simulink model "DYNctl_ver4_etud_obfusc"  (R2021b)
settings: Solver=ode45  StartTime=0.0  StopTime=tfin  FixedStep=0.001  RelTol=1e-09  EnableMultiTasking=on
values from neighbouring files (symbols this model uses):
  A_lineaire = [ ... (first row only)    [equation_lineaire.m]
  Ax_e = 0    [Valeur_Equilibre.m]
  Ay_e = 0    [Valeur_Equilibre.m]
  B_lineaire = [ ... (first row only)    [equation_lineaire.m]
  C_lineaire = [ ... (first row only)    [equation_lineaire.m]
  C_variable_etat = eye(13,13)    [equation_lineaire.m]
  D_lineaire = zeros(7,3)    [equation_lineaire.m]
  D_variable_etat = zeros(13,3)    [equation_lineaire.m]
  Ia_e = i_A    [Valeur_Equilibre.m]
  Ib_e = i_B    [Valeur_Equilibre.m]
  Ic_e = i_C    [Valeur_Equilibre.m]
  Px_e = Px_sphere    [Valeur_Equilibre.m]
  Py_e = Py_sphere    [Valeur_Equilibre.m]
  Pz_e = Pz_plaque    [Valeur_Equilibre.m]
  Va_e = RR*Ia_e    [Valeur_Equilibre.m]
  Vb_e = RR*Ib_e    [Valeur_Equilibre.m]
  Vc_e = RR*Ic_e    [Valeur_Equilibre.m]
  Vx_e = 0    [Valeur_Equilibre.m]
  Vy_e = 0    [Valeur_Equilibre.m]
  Vz_e = 0    [Valeur_Equilibre.m]
  Wx_e = 0    [Valeur_Equilibre.m]
  Wy_e = 0    [Valeur_Equilibre.m]
  zD_e = Pz_plaque - XD*Ay_eq + YD*Ax_eq    [Valeur_Equilibre.m]
  zE_e = Pz_plaque - XE*Ay_eq + YE*Ax_eq    [Valeur_Equilibre.m]
  zF_e = Pz_plaque - XF*Ay_eq + YF*Ax_eq    [Valeur_Equilibre.m]
settings Model: Creator=delafontaine  LastModifiedBy=alexi
settings SolverCC: AlgebraicLoopSolver=LineSearch
settings DataIOCC: LimitDataPoints=on  SaveFormat=Array  SignalLoggingSaveFormat=ModelDataLogs  ReturnWorkspaceOutputs=off
settings OptimizationCC: LifeSpan=inf
settings DebuggingCC: UnderspecifiedInitializationDetection=Classic  MergeDetectMultiDrivingBlocksExec=none  MultiTaskDSMMsg=warning  MultiTaskCondExecSysMsg=none  SFUnexpectedBacktrackingDiag=warning  SFNoUnconditionalDefaultTransitionDiag=warning  SFExecutionAtInitializationDiag=none  SFMachineParentedDataDiag=warning  ArithmeticOperatorsInVariantConditions=warning
settings HardwareCC: ProdBitPerPointer=32  ProdBitPerSizeT=32  ProdBitPerPtrDiffT=32  ProdLargestAtomicFloat=None  ProdIntDivRoundTo=Undefined  ProdEndianess=Unspecified  ProdWordSize=32  ProdHWDeviceType=32-bit Generic
settings ModelReferenceCC: PropagateSignalLabelsOutOfModel=off
settings SFSimCC: SimUseLocalCustomCode=off  CustomCodeUndefinedFunction=UseInterfaceOnly
settings RTWCC: RTWUseLocalCustomCode=off
settings CodeAppCC: StateflowObjectComments=on
settings GRTTargetCC: TargetLangStandard=C89/C90 (ANSI)
settings ConfigComp: CovMetricSettings=dw  CovSaveCumulativeToWorkspaceVar=on  CovSaveSingleToWorkspaceVar=on  CovExternalEMLEnable=off  CovSFcnEnable=off

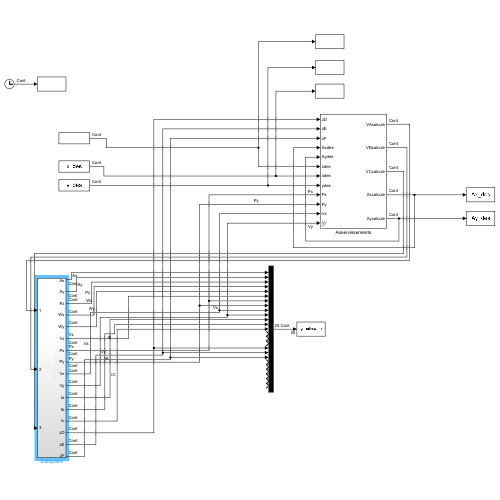
[thumbnail: Simulink's stored preview of the top-level diagram]
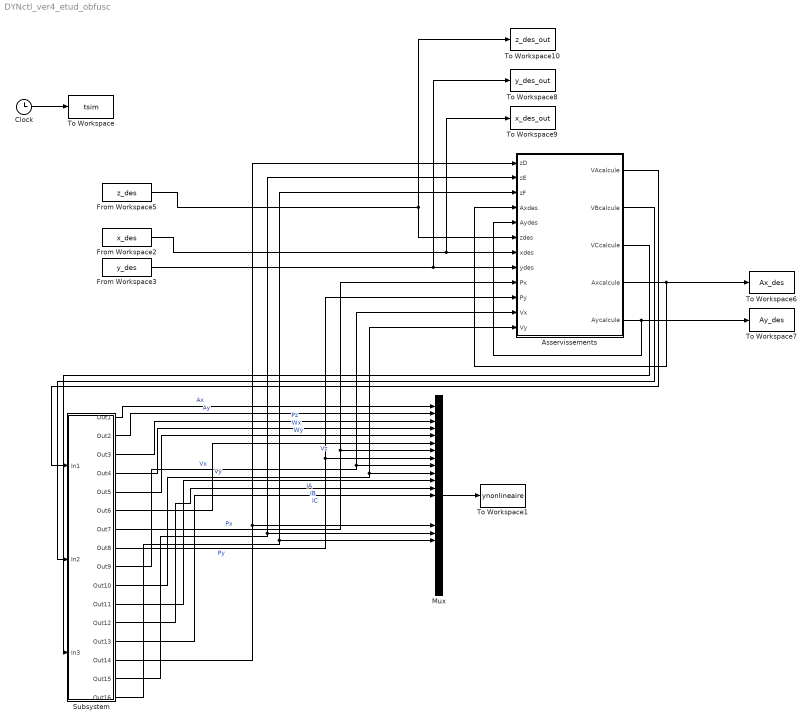
== system DYNctl_ver4_etud_obfusc ==
  Asservissements : Subsystem
      mask help: Simulink:masks:GenSFuncDesc_MD
      mask Help: eval('feval(''rtwprivate'',''rtwhelpview'',''rtw_sfcn_block'')');
  Clock : Clock
  From Workspace2 : FromWorkspace  VariableName=x_des  Interpolate=off  OutputAfterFinalValue=Holding final value
  From Workspace3 : FromWorkspace  VariableName=y_des  Interpolate=off  OutputAfterFinalValue=Holding final value
  From Workspace5 : FromWorkspace  VariableName=z_des  Interpolate=off  OutputAfterFinalValue=Holding final value
  Mux : Mux  Inputs=25
  Subsystem : Subsystem
  To Workspace : ToWorkspace  VariableName=tsim  SampleTime=-1
  To Workspace1 : ToWorkspace  VariableName=ynonlineaire  SampleTime=-1
  To Workspace10 : ToWorkspace  VariableName=z_des_out  SampleTime=-1
  To Workspace6 : ToWorkspace  VariableName=Ax_des  SampleTime=-1
  To Workspace7 : ToWorkspace  VariableName=Ay_des  SampleTime=-1
  To Workspace8 : ToWorkspace  VariableName=y_des_out  SampleTime=-1
  To Workspace9 : ToWorkspace  VariableName=x_des_out  SampleTime=-1
  wires:
  Mux/1 -> To Workspace1/1
  Clock/1 -> To Workspace/1
  From Workspace5/1 -> Asservissements/6(zdes), To Workspace10/1
  Subsystem/1(Out1) -> Mux/1  "Ax"
  Subsystem/2(Out2) -> Mux/2  "Ay"
  Subsystem/3(Out3) -> Mux/3  "Pz"
  Subsystem/4(Out4) -> Mux/4  "Wx"
  Subsystem/5(Out5) -> Mux/5  "Wy"
  Subsystem/6(Out6) -> Mux/6  "Vz"
  Subsystem/7(Out7) -> Asservissements/9(Px), Mux/7  "Px"
  Subsystem/8(Out8) -> Asservissements/10(Py), Mux/8  "Py"
  Subsystem/9(Out9) -> Asservissements/11(Vx), Mux/9  "Vx"
  Subsystem/10(Out10) -> Asservissements/12(Vy), Mux/10  "Vy"
  Subsystem/11(Out11) -> Mux/11  "IA"
  Subsystem/12(Out12) -> Mux/12  "IB"
  Subsystem/13(Out13) -> Mux/13  "IC"
  From Workspace3/1 -> Asservissements/8(ydes), To Workspace8/1
  From Workspace2/1 -> Asservissements/7(xdes), To Workspace9/1
  Subsystem/14(Out14) -> Asservissements/1(zD), Mux/17
  Subsystem/15(Out15) -> Asservissements/2(zE), Mux/18
  Subsystem/16(Out16) -> Asservissements/3(zF), Mux/19
  Asservissements/4(Axcalcule) -> Asservissements/4(Axdes), To Workspace6/1
  Asservissements/5(Aycalcule) -> Asservissements/5(Aydes), To Workspace7/1
  Asservissements/1(VAcalcule) -> Subsystem/1(In1)
  Asservissements/2(VBcalcule) -> Subsystem/2(In2)
  Asservissements/3(VCcalcule) -> Subsystem/3(In3)

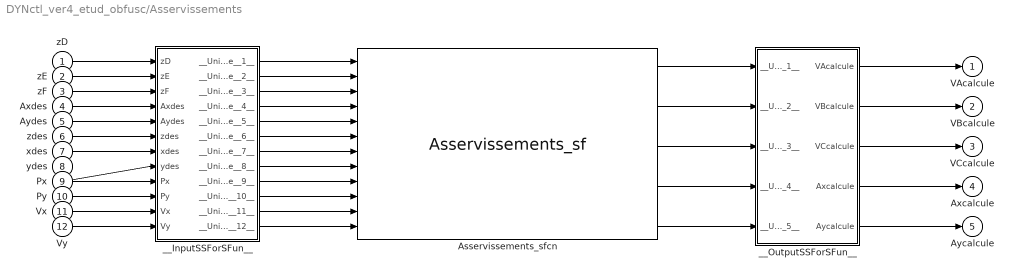
== system DYNctl_ver4_etud_obfusc/Asservissements ==
  zD : Inport
  zE : Inport  Port=2
  zF : Inport  Port=3
  Axdes : Inport  Port=4
  Aydes : Inport  Port=5
  zdes : Inport  Port=6
  xdes : Inport  Port=7
  ydes : Inport  Port=8
  Px : Inport  Port=9
  Py : Inport  Port=10
  Vx : Inport  Port=11
  Vy : Inport  Port=12
  Asservissements_sfcn : S-Function  FunctionName=Asservissements_sf  SFunctionModules=""  SFunctionDeploymentMode=off  EnableBusSupport=off  mask{rtw_sf_name=Asservissements_sf, showVar=off}
      mask prompts: rtw_sf_name "Simulink:masks:GenSFuncName_MP"; showVar "Simulink:masks:GenSFuncShowModuleList_MP"
      mask help: Simulink:masks:GenSFuncDesc_MD
      mask init:
      | displist = '';
      | if ~strcmp(get_param(gcb, 'FunctionName'), rtw_sf_name);
      |   set_param(gcb, 'FunctionName', rtw_sf_name);
      | end
      | % Check if we are generating code
      | rtw_mode = false;
      | if strcmpi(get_param(bdroot(gcb),'SimulationStatus'),'Initializing')
      | 	rtw_mode = strcmpi(get_param(bdroot(gcb),'BuildingRTWCode'),'on') && ...
      | 		~strcmpi(get_param(bdroot(gcb),'TargetStyle'),'SimulationTarget');
      | end
      | if showVar || rtw_mode
      | 	if exist('rtwsfunc') == 2 | exist('rtwsfunc') == 6
      | 		tmplist = rtwsfunc(rtw_sf_name,gcb);
      | 		tmplist = DAStudio.message('Simulink:masks:GenSFuncListOfModules_IC', tmplist);
      | 	elseif showVar
      | 		tmplist1 = DAStudio.message('Simulink:masks:GenSFuncListOfModules_IC', '');
      |         tmplist2 = DAStudio.message('Simulink:masks:GenSFuncNotLicensed_IC');
      |         tmplist = [tmplist1 tmplist2];
      |  	end
      | end
      | if showVar
      |   displist = tmplist;
      | end
      settings: CopyFcn=|
      | if ~strcmp(get_param(gcb,'Linkstatus'),'none') && ...
      | ~strcmp(get_param(gcb,'Linkstatus'),'implicit')
      |   set_param(gcb,'LinkStatus','none');
      | end
      mask Help: eval('feval(''rtwprivate'',''rtwhelpview'',''rtw_sfcn_block'')');
      mask Display:
      | port_label('input',1,'zD');
      | port_label('input',2,'zE');
      | port_label('input',3,'zF');
      | port_label('input',4,'Axdes');
      | port_label('input',5,'Aydes');
      | port_label('input',6,'zdes');
      | port_label('input',7,'xdes');
      | port_label('input',8,'ydes');
      | port_label('input',9,'Px');
      | port_label('input',10,'Py');
      | port_label('input',11,'Vx');
      | port_label('input',12,'Vy');
      | port_label('output',1,'VAcalcule');
      | port_label('output',2,'VBcalcule');
      | port_label('output',3,'VCcalcule');
      | port_label('output',4,'Axcalcule');
      | port_label('output',5,'Aycalcule');
  __InputSSForSFun__ : Subsystem
  __OutputSSForSFun__ : Subsystem
  VAcalcule : Outport
  VBcalcule : Outport  Port=2
  VCcalcule : Outport  Port=3
  Axcalcule : Outport  Port=4
  Aycalcule : Outport  Port=5
  wires:
  zD/1 -> __InputSSForSFun__/1(zD)
  zE/1 -> __InputSSForSFun__/2(zE)
  zF/1 -> __InputSSForSFun__/3(zF)
  Axdes/1 -> __InputSSForSFun__/4(Axdes)
  Aydes/1 -> __InputSSForSFun__/5(Aydes)
  zdes/1 -> __InputSSForSFun__/6(zdes)
  xdes/1 -> __InputSSForSFun__/7(xdes)
  ydes/1 -> __InputSSForSFun__/8(ydes)
  Px/1 -> __InputSSForSFun__/9(Px)
  Py/1 -> __InputSSForSFun__/10(Py)
  Vx/1 -> __InputSSForSFun__/11(Vx)
  Vy/1 -> __InputSSForSFun__/12(Vy)
  __InputSSForSFun__/1(__UniqueOutportName__1__) -> Asservissements_sfcn/1
  __InputSSForSFun__/2(__UniqueOutportName__2__) -> Asservissements_sfcn/2
  __InputSSForSFun__/3(__UniqueOutportName__3__) -> Asservissements_sfcn/3
  __InputSSForSFun__/4(__UniqueOutportName__4__) -> Asservissements_sfcn/4
  __InputSSForSFun__/5(__UniqueOutportName__5__) -> Asservissements_sfcn/5
  __InputSSForSFun__/6(__UniqueOutportName__6__) -> Asservissements_sfcn/6
  __InputSSForSFun__/7(__UniqueOutportName__7__) -> Asservissements_sfcn/7
  __InputSSForSFun__/8(__UniqueOutportName__8__) -> Asservissements_sfcn/8
  __InputSSForSFun__/9(__UniqueOutportName__9__) -> Asservissements_sfcn/9
  __InputSSForSFun__/10(__UniqueOutportName__10__) -> Asservissements_sfcn/10
  __InputSSForSFun__/11(__UniqueOutportName__11__) -> Asservissements_sfcn/11
  __InputSSForSFun__/12(__UniqueOutportName__12__) -> Asservissements_sfcn/12
  Asservissements_sfcn/1 -> __OutputSSForSFun__/1(__UniqueInportName__1__)
  Asservissements_sfcn/2 -> __OutputSSForSFun__/2(__UniqueInportName__2__)
  Asservissements_sfcn/3 -> __OutputSSForSFun__/3(__UniqueInportName__3__)
  Asservissements_sfcn/4 -> __OutputSSForSFun__/4(__UniqueInportName__4__)
  Asservissements_sfcn/5 -> __OutputSSForSFun__/5(__UniqueInportName__5__)
  __OutputSSForSFun__/1(VAcalcule) -> VAcalcule/1
  __OutputSSForSFun__/2(VBcalcule) -> VBcalcule/1
  __OutputSSForSFun__/3(VCcalcule) -> VCcalcule/1
  __OutputSSForSFun__/4(Axcalcule) -> Axcalcule/1
  __OutputSSForSFun__/5(Aycalcule) -> Aycalcule/1

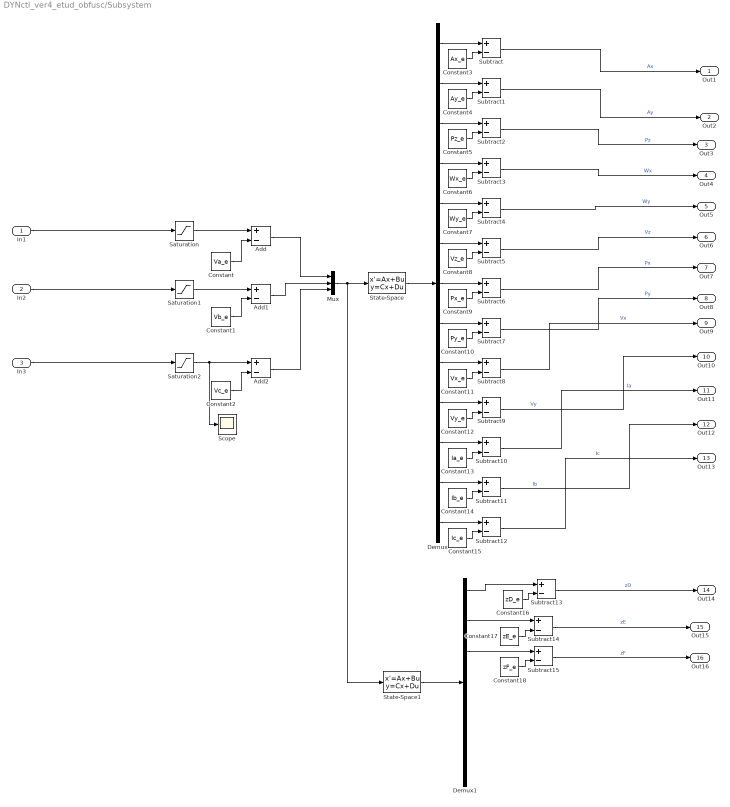
== system DYNctl_ver4_etud_obfusc/Subsystem ==
  In1 : Inport
  In2 : Inport  Port=2
  In3 : Inport  Port=3
  Add : Sum  Inputs=+-
  Add1 : Sum  Inputs=+-
  Add2 : Sum  Inputs=+-
  Constant : Constant  Value=Va_e
  Constant1 : Constant  Value=Vb_e
  Constant10 : Constant  Value=Py_e
  Constant11 : Constant  Value=Vx_e
  Constant12 : Constant  Value=Vy_e
  Constant13 : Constant  Value=Ia_e
  Constant14 : Constant  Value=Ib_e
  Constant15 : Constant  Value=Ic_e
  Constant16 : Constant  Value=zD_e
  Constant17 : Constant  Value=zE_e
  Constant18 : Constant  Value=zF_e
  Constant2 : Constant  Value=Vc_e
  Constant3 : Constant  Value=Ax_e
  Constant4 : Constant  Value=Ay_e
  Constant5 : Constant  Value=Pz_e
  Constant6 : Constant  Value=Wx_e
  Constant7 : Constant  Value=Wy_e
  Constant8 : Constant  Value=Vz_e
  Constant9 : Constant  Value=Px_e
  Demux : Demux  Outputs=13
  Demux1 : Demux  Outputs=7
  Mux : Mux  Inputs=3
  Saturation : Saturate  UpperLimit=22  LowerLimit=-22
  Saturation1 : Saturate  UpperLimit=22  LowerLimit=-22
  Saturation2 : Saturate  UpperLimit=22  LowerLimit=-22
  Scope : Scope
  State-Space : StateSpace  A=A_lineaire  B=B_lineaire  C=C_variable_etat  D=D_variable_etat  InitialCondition=0
  State-Space1 : StateSpace  A=A_lineaire  B=B_lineaire  C=C_lineaire  D=D_lineaire  InitialCondition=0
  Subtract{,1..15} (16 alike) : Sum  Inputs=+-
  Out1 : Outport
  Out2 : Outport  Port=2
  Out3 : Outport  Port=3
  Out4 : Outport  Port=4
  Out5 : Outport  Port=5
  Out6 : Outport  Port=6
  Out7 : Outport  Port=7
  Out8 : Outport  Port=8
  Out9 : Outport  Port=9
  Out10 : Outport  Port=10
  Out11 : Outport  Port=11
  Out12 : Outport  Port=12
  Out13 : Outport  Port=13
  Out14 : Outport  Port=14
  Out15 : Outport  Port=15
  Out16 : Outport  Port=16
  wires:
  Constant7/1 -> Subtract4/2
  Saturation2/1 -> Scope/1, Add2/1
  Demux/7 -> Subtract6/1
  Subtract/1 -> Out1/1  "Ax"
  State-Space/1 -> Demux/1
  Subtract8/1 -> Out9/1  "Vx"
  Subtract10/1 -> Out11/1  "Ia"
  Demux/5 -> Subtract4/1
  Subtract4/1 -> Out5/1  "Wy"
  Constant4/1 -> Subtract1/2
  Subtract2/1 -> Out3/1  "Pz"
  Constant15/1 -> Subtract12/2
  Demux/3 -> Subtract2/1
  Demux/8 -> Subtract7/1
  Constant11/1 -> Subtract8/2
  Constant2/1 -> Add2/2
  Constant13/1 -> Subtract10/2
  Constant5/1 -> Subtract2/2
  In2/1 -> Saturation1/1
  Demux/11 -> Subtract10/1
  Demux/6 -> Subtract5/1
  Demux/4 -> Subtract3/1
  Constant8/1 -> Subtract5/2
  Demux/9 -> Subtract8/1
  Saturation/1 -> Add/1
  Constant/1 -> Add/2
  Add2/1 -> Mux/3
  Subtract12/1 -> Out13/1  "Ic"
  Mux/1 -> State-Space1/1, State-Space/1
  Demux/1 -> Subtract/1
  Subtract11/1 -> Out12/1  "Ib"
  Constant1/1 -> Add1/2
  Demux/2 -> Subtract1/1
  Add1/1 -> Mux/2
  Demux/12 -> Subtract11/1
  Constant3/1 -> Subtract/2
  Constant10/1 -> Subtract7/2
  Constant12/1 -> Subtract9/2
  Subtract5/1 -> Out6/1  "Vz"
  Demux/10 -> Subtract9/1
  Constant6/1 -> Subtract3/2
  Demux/13 -> Subtract12/1
  Subtract9/1 -> Out10/1  "Vy"
  Constant9/1 -> Subtract6/2
  Saturation1/1 -> Add1/1
  Constant14/1 -> Subtract11/2
  Add/1 -> Mux/1
  In3/1 -> Saturation2/1
  Subtract7/1 -> Out8/1  "Py"
  Subtract3/1 -> Out4/1  "Wx"
  Subtract1/1 -> Out2/1  "Ay"
  Subtract6/1 -> Out7/1  "Px"
  In1/1 -> Saturation/1
  State-Space1/1 -> Demux1/1
  Demux1/1 -> Subtract13/1
  Constant16/1 -> Subtract13/2
  Constant17/1 -> Subtract14/2
  Demux1/2 -> Subtract14/1
  Demux1/3 -> Subtract15/1
  Constant18/1 -> Subtract15/2
  Subtract13/1 -> Out14/1  "zD"
  Subtract14/1 -> Out15/1  "zE"
  Subtract15/1 -> Out16/1  "zF"

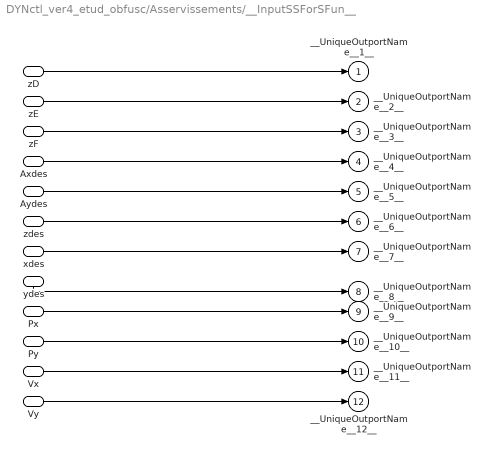
== system DYNctl_ver4_etud_obfusc/Asservissements/__InputSSForSFun__ ==
  zD : Inport
  zE : Inport  Port=2
  zF : Inport  Port=3
  Axdes : Inport  Port=4
  Aydes : Inport  Port=5
  zdes : Inport  Port=6
  xdes : Inport  Port=7
  ydes : Inport  Port=8
  Px : Inport  Port=9
  Py : Inport  Port=10
  Vx : Inport  Port=11
  Vy : Inport  Port=12
  __UniqueOutportName__1__ : Outport
  __UniqueOutportName__2__ : Outport  Port=2
  __UniqueOutportName__3__ : Outport  Port=3
  __UniqueOutportName__4__ : Outport  Port=4
  __UniqueOutportName__5__ : Outport  Port=5
  __UniqueOutportName__6__ : Outport  Port=6
  __UniqueOutportName__7__ : Outport  Port=7
  __UniqueOutportName__8__ : Outport  Port=8
  __UniqueOutportName__9__ : Outport  Port=9
  __UniqueOutportName__10__ : Outport  Port=10
  __UniqueOutportName__11__ : Outport  Port=11
  __UniqueOutportName__12__ : Outport  Port=12
  wires:
  zD/1 -> __UniqueOutportName__1__/1
  zE/1 -> __UniqueOutportName__2__/1
  zF/1 -> __UniqueOutportName__3__/1
  Axdes/1 -> __UniqueOutportName__4__/1
  Aydes/1 -> __UniqueOutportName__5__/1
  zdes/1 -> __UniqueOutportName__6__/1
  xdes/1 -> __UniqueOutportName__7__/1
  ydes/1 -> __UniqueOutportName__8__/1
  Px/1 -> __UniqueOutportName__9__/1
  Py/1 -> __UniqueOutportName__10__/1
  Vx/1 -> __UniqueOutportName__11__/1
  Vy/1 -> __UniqueOutportName__12__/1

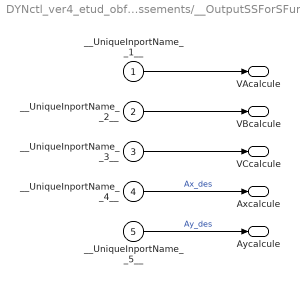
== system DYNctl_ver4_etud_obfusc/Asservissements/__OutputSSForSFun__ ==
  __UniqueInportName__1__ : Inport
  __UniqueInportName__2__ : Inport  Port=2
  __UniqueInportName__3__ : Inport  Port=3
  __UniqueInportName__4__ : Inport  Port=4
  __UniqueInportName__5__ : Inport  Port=5
  VAcalcule : Outport
  VBcalcule : Outport  Port=2
  VCcalcule : Outport  Port=3
  Axcalcule : Outport  Port=4
  Aycalcule : Outport  Port=5
  wires:
  __UniqueInportName__1__/1 -> VAcalcule/1
  __UniqueInportName__2__/1 -> VBcalcule/1
  __UniqueInportName__3__/1 -> VCcalcule/1
  __UniqueInportName__4__/1 -> Axcalcule/1  "Ax_des"
  __UniqueInportName__5__/1 -> Aycalcule/1  "Ay_des"
